simulink library "medusa5h1_stereo"  (R2022b)
settings: Solver=VariableStepAuto  StartTime=0.0  StopTime=10.0  RelTol=1e-3
values from neighbouring files (symbols this model uses):
  MedusaConfig = struct('BandSplitConfig', BandSplitConfig,                            'DRFDPConfig', DRFDPConfig,                            'FRFDPConfig', FRFDPConfig,                            'SurroundConfig', SurroundConfig,                            'MSConfig', MSConfig,                            'PremixConfig', PremixConfig.Stereo,                            'PremixTune', PremixTune.Stereo,               ...(+1303 chars)    [medusa5h1_init.m]
undefined symbols (not defined in the file or in its folder): Config, MedusaBTC, Row, VLSConfig
libraries: TuneVar x25, MedusaDelays x19, FeaturePath x15, RTC x6, MedusaCaeEnable x4, MedusaDrHoligramEq x4, TOP x4, BassManager x2, StateVar x2, TrebleBoost x2, dspstat3 x2, MedusaBandSplit x2
(part 2 of 2)

== system medusa5h1_stereo/Medusa + Holigram/Medusa5H1 Part 5/Triggered Subsystem ==
  Trigger : TriggerPort  TriggerType=function-call  VariantControl=(inherit)
  Constant : Constant  Value=0
  Data Store Write : DataStoreWrite  DataStoreName=MedusaOverheadHoligramEnable  IndexOptions=Index vector (dialog)  Indices=1  OutputSizes=1
  wires:
  Constant/1 -> Data Store Write/1

== system medusa5h1_stereo/Medusa + Holigram/Medusa5H1 Part 6/Speaker Delay Tune ==
  Output Delay Translation with Headrest : MedusaDelays/HeadrestOutputDelayTranslation  Config=ConfigBTC.HeadrestOutputDelayTranslation
  TOP3 : TOP/TOP  TriggerInit=[645 305 895 365]  TopName=FRSpeakerDelay  DataTypeOut=int32  BankNumber=0  PreOverlay=false  PostOverlay=false  Role=Automatic
      settings: SourceProductName=Bose Talaria
  TOP5 : TOP/TOP  TriggerInit=[645 155 895 215]  TopName=DRSpeakerDelay  DataTypeOut=int32  BankNumber=0  PreOverlay=false  PostOverlay=false  Role=Automatic
      settings: SourceProductName=Bose Talaria
  Tune Variable : TuneVar/TuneVar  TuneName=HeadrestDrvSpeakerDelaySamples  SpecifyMaxSize=off  VariableDim=1 (Row)  MaxSize=[1 1]  TunabilityNumber=1  MinValue=[]  MaxValue=[]  TriggerInit=[20 195 245 245]  MaskValue=[0]
      settings: SourceProductName=Bose Talaria
  Tune Variable1 : TuneVar/TuneVar  TuneName=NonHeadrestSpeakerDelaySamples  SpecifyMaxSize=off  VariableDim=1 (Row)  MaxSize=[]  TunabilityNumber=1  MinValue=[]  MaxValue=[]  TriggerInit=[20 120 245 170]  MaskValue=HRDelayConfig.DRNonHRDelay
      settings: SourceProductName=Bose Talaria
  Tune Variable4 : TuneVar/TuneVar  TuneName=HeadrestPaxSpeakerDelaySamples  SpecifyMaxSize=off  VariableDim=1 (Row)  MaxSize=[1 1]  TunabilityNumber=1  MinValue=[]  MaxValue=[]  TriggerInit=[20 270 245 320]  MaskValue=[0]
      settings: SourceProductName=Bose Talaria
  Tune Variable5 : TuneVar/TuneVar  TuneName=FRHoligramDelaySamples  SpecifyMaxSize=off  VariableDim=1 (Row)  MaxSize=[]  TunabilityNumber=1  MinValue=[]  MaxValue=[]  TriggerInit=[20 345 245 395]  MaskValue=HRDelayConfig.FRSpkrDelay
      settings: SourceProductName=Bose Talaria
  DRSpeakerDelay : Outport
  FRSpeakerDelay : Outport  Port=2
  wires:
  TOP5/1 -> DRSpeakerDelay/1  "DRSpeakerDelay"
  TOP3/1 -> FRSpeakerDelay/1  "FRSpeakerDelay"
  Tune Variable1/1 -> Output Delay Translation with Headrest/1  "NonHeadrestSpeakerDelaySamples"
  Tune Variable/1 -> Output Delay Translation with Headrest/2  "HeadrestDrvSpeakerDelaySamples"
  Tune Variable4/1 -> Output Delay Translation with Headrest/3  "HeadrestPaxSpeakerDelaySamples"
  Tune Variable5/1 -> Output Delay Translation with Headrest/4  "FRHoligramDelaySamples"
  Output Delay Translation with Headrest/1 -> TOP5/1
  Output Delay Translation with Headrest/2 -> TOP3/1

== system medusa5h1_stereo/Medusa5H1 Stereo/Medusa5H1 Part 1/CAE Treble Boost ==
  note: 1) Add Subsystem or Model blocks as valid variant choices.
      | 2) You cannot connect blocks at this level. At simulation, connectivity is automatically
      | determined, based on the active variant and port name matching.
  AudioIn : Inport
  Audio Passthrough : Subsystem  VariantControl=include_CAE == 0
  CAE Treble Boost : Subsystem  VariantControl=include_CAE == 1
  Out : Outport
  CAEEnable : Outport  Port=2

== system medusa5h1_stereo/Medusa5H1 Stereo/Medusa5H1 Part 2/Alignment Delay ==
  LRhp : Inport
  Full-rate Alignment Delay Translation : MedusaDelays/MedusaFullRateAlignmentDelayTranslation  Config=Config.TrebleDelayTranslation
  Treble Delay : MedusaDelays/MedusaAlignmentDelay  Config=Config.TrebleDelay
  Tune Variable1 : TuneVar/TuneVar  TuneName=DeciRateNearWiggleFilterDelaySamples  SpecifyMaxSize=off  VariableDim=1 (Row)  MaxSize=[1 1]  TunabilityNumber=1  MinValue=[]  MaxValue=[]  TriggerInit=[-55 450 110 500]  MaskValue=Config.TrebleDelayTranslation.DefaultTuning.DeciRateNearWiggleDelay
      settings: SourceProductName=Bose Talaria
  Tune Variable4 : TuneVar/TuneVar  TuneName=DeciRateWiggleFilterDelaySamples  SpecifyMaxSize=off  VariableDim=1 (Row)  MaxSize=[1 1]  TunabilityNumber=1  MinValue=[]  MaxValue=[]  TriggerInit=[-55 385 110 435]  MaskValue=Config.TrebleDelayTranslation.DefaultTuning.DeciRateWiggleDelay
      settings: SourceProductName=Bose Talaria
  Tune Variable5 : TuneVar/TuneVar  TuneName=HoligramFilterAlignmentDelaySamples  SpecifyMaxSize=off  VariableDim=1 (Row)  MaxSize=[1 1]  TunabilityNumber=1  MinValue=[]  MaxValue=[]  TriggerInit=[-55 515 110 565]  MaskValue=Config.TrebleDelayTranslation.DefaultTuning.HoligramDelay
      settings: SourceProductName=Bose Talaria
  LRtreble : Outport
  wires:
  [TrebleDelay] -> Treble Delay/2
  Tune Variable4/1 -> Full-rate Alignment Delay Translation/1  "DeciRateWiggleFilterDelaySamples"
  Full-rate Alignment Delay Translation/1 -> [TrebleDelay]
  Treble Delay/1 -> LRtreble/1  "LRtreble"
  LRhp/1 -> Treble Delay/1
  Tune Variable5/1 -> Full-rate Alignment Delay Translation/3  "HoligramFilterAlignmentDelaySamples"
  Tune Variable1/1 -> Full-rate Alignment Delay Translation/2  "DeciRateNearWiggleFilterDelaySamples"

== system medusa5h1_stereo/Medusa5H1 Stereo/Medusa5H1 Part 3/Bypass ==
  Action Port : ActionPort
  Constant : Constant  Value=zeros(config.PremixConfig.frame_size, config.PremixConfig.NumPremixOut)  OutDataTypeStr=single
  Constant1 : Constant  Value=Config.DefaultFullRateMixerOutput  OutDataTypeStr=single
  PremixOut : Outport  VectorParamsAs1DForOutWhenUnconnected=off
  FRMixerOut : Outport  Port=2  VectorParamsAs1DForOutWhenUnconnected=off
  wires:
  Constant/1 -> PremixOut/1
  Constant1/1 -> FRMixerOut/1

== system medusa5h1_stereo/Medusa5H1 Stereo/Medusa5H1 Part 3/Enable State Write ==
  Trigger : TriggerPort  TriggerType=function-call  VariantControl=Variant  PortDimensions=1
  Constant : Constant  Value=0  OutDataTypeStr=uint32
  Data Store Write : DataStoreWrite  DataStoreName=MedusaPostUpmixEnable  IndexOptions=Index vector (dialog)  Indices=1  OutputSizes=1
  wires:
  Constant/1 -> Data Store Write/1

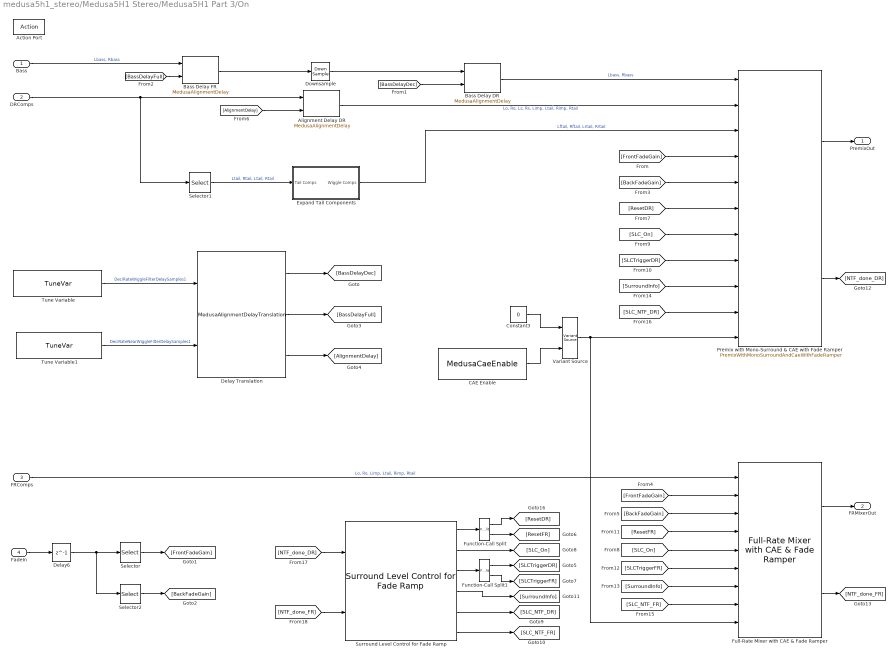
== system medusa5h1_stereo/Medusa5H1 Stereo/Medusa5H1 Part 3/On ==
  Bass : Inport  OutDataTypeStr=single
  DRComps : Inport  Port=2  OutDataTypeStr=single
  FRComps : Inport  Port=3  OutDataTypeStr=single
  FadeIn : Inport  Port=4  OutDataTypeStr=single
  Action Port : ActionPort
  Alignment Delay DR : MedusaDelays/MedusaAlignmentDelay  Config=Config.MidrangeDelay
  Bass Delay DR : MedusaDelays/MedusaAlignmentDelay  Config=Config.DeciRateBassDelay
  Bass Delay FR : MedusaDelays/MedusaAlignmentDelay  Config=Config.FullRateBassDelay
  CAE Enable : MedusaCaeEnable/MedusaCaeEnable  Config=Config.PremixCaeEnable  MaskMessageName=PremixCAEEnable
  Constant3 : Constant  Value=0  OutDataTypeStr=int32  SampleTime=-1
  Delay Translation : MedusaDelays/MedusaAlignmentDelayTranslation  Config=Config.AlignmentDelayTranslation
  Delay6 : Delay  DelayLength=1
  Downsample : DownSample  N=4
  Expand Tail Components : Subsystem  TreatAsAtomicUnit=on  RTWFileName=MedusaExpandTailComps
      settings: RTWSystemCode=Nonreusable function  RTWFileNameOpts=User specified  FunctionWithSeparateData=on
  Full-Rate Mixer with CAE & Fade Ramper : MedusaFullRateMixer/Full-Rate Mixer with CAE & Fade Ramper  MedusaFRMConfig=config.FRMConfig  MedusaFRMTune=config.FRMTune
  Function-Call Split : FunctionCallSplit  IconShape=distinctive  NumOutputPorts=2  OutputPortLayout=default
  Function-Call Split1 : FunctionCallSplit  IconShape=distinctive  NumOutputPorts=2  OutputPortLayout=default
  Premix with Mono-Surround & CAE with Fade Ramper : MedusaPremix/PremixWithMonoSurroundAndCaeWithFadeRamper  MedusaPremixConfig=config.PremixConfig  MedusaPremixTune=config.PremixTune  MSConfig=config.MSConfig
  Selector : Selector  NumberOfDimensions=2  InputPortWidth=2  IndexOptions=Index vector (dialog),Index vector (dialog)  Indices=1,1  OutputSizes=1,1
  Selector1 : Selector  NumberOfDimensions=2  InputPortWidth=3  IndexOptions=Select all,Index vector (dialog)  Indices=[1 3],[6 8 6 8]  OutputSizes=1,1
  Selector2 : Selector  NumberOfDimensions=2  InputPortWidth=2  IndexOptions=Index vector (dialog),Index vector (dialog)  Indices=1,2  OutputSizes=1,1
  Surround Level Control for Fade Ramp : MedusaSurroundLevelControl/Surround Level Control for Fade Ramp  SurroundConfig=config.SurroundConfig
  Tune Variable : TuneVar/TuneVar  TuneName=DeciRateWiggleFilterDelaySamples1  SpecifyMaxSize=off  VariableDim=1 (Row)  MaxSize=[1 1]  TunabilityNumber=1  MinValue=[]  MaxValue=[]  TriggerInit=[-70 585 100 635]  MaskValue=Config.AlignmentDelayTranslation.DefaultTuning.DeciRateWiggleDelay
      settings: SourceProductName=Bose Talaria
  Tune Variable1 : TuneVar/TuneVar  TuneName=DeciRateNearWiggleFilterDelaySamples1  SpecifyMaxSize=off  VariableDim=1 (Row)  MaxSize=[1 1]  TunabilityNumber=1  MinValue=[]  MaxValue=[]  TriggerInit=[-65 705 100 755]  MaskValue=Config.AlignmentDelayTranslation.DefaultTuning.DeciRateNearWiggleDelay
      settings: SourceProductName=Bose Talaria
  Variant Source : VariantSource
  PremixOut : Outport  VectorParamsAs1DForOutWhenUnconnected=off
  FRMixerOut : Outport  Port=2  VectorParamsAs1DForOutWhenUnconnected=off
  wires:
  Selector/1 -> [FrontFadeGain]
  Delay6/1 -> Selector/1, Selector2/1
  Selector2/1 -> [BackFadeGain]
  FadeIn/1 -> Delay6/1
  Bass Delay FR/1 -> Downsample/1
  Alignment Delay DR/1 -> Premix with Mono-Surround & CAE with Fade Ramper/2  "Lo, Ro, Ls, Rs, Limp, Ltail, Rimp, Rtail"
  DRComps/1 -> Selector1/1, Alignment Delay DR/1
  Selector1/1 -> Expand Tail Components/1(Tail Comps)  "Ltail, Rtail, Ltail, Rtail"
  Bass/1 -> Bass Delay FR/1  "Lbass, Rbass"
  Expand Tail Components/1(Wiggle Comps) -> Premix with Mono-Surround & CAE with Fade Ramper/3  "Lftail, Rftail, Lrtail, Rrtail"
  [BackFadeGain] -> Premix with Mono-Surround & CAE with Fade Ramper/5
  [FrontFadeGain] -> Full-Rate Mixer with CAE & Fade Ramper/2
  Premix with Mono-Surround & CAE with Fade Ramper/1 -> PremixOut/1
  [BackFadeGain] -> Full-Rate Mixer with CAE & Fade Ramper/3
  Full-Rate Mixer with CAE & Fade Ramper/1 -> FRMixerOut/1
  [FrontFadeGain] -> Premix with Mono-Surround & CAE with Fade Ramper/4
  Delay Translation/3 -> [AlignmentDelay]
  Delay Translation/2 -> [BassDelayFull]
  Delay Translation/1 -> [BassDelayDec]
  Tune Variable/1 -> Delay Translation/1  "DeciRateWiggleFilterDelaySamples1"
  [BassDelayFull] -> Bass Delay FR/2
  [AlignmentDelay] -> Alignment Delay DR/2
  Bass Delay DR/1 -> Premix with Mono-Surround & CAE with Fade Ramper/1  "Lbass, Rbass"
  [BassDelayDec] -> Bass Delay DR/2
  Downsample/1 -> Bass Delay DR/1
  FRComps/1 -> Full-Rate Mixer with CAE & Fade Ramper/1  "Lo, Ro, Limp, Ltail, Rimp, Rtail"
  Surround Level Control for Fade Ramp/1 -> Function-Call Split/1
  Surround Level Control for Fade Ramp/3 -> Function-Call Split1/1
  Function-Call Split/1 -> [ResetDR]
  Function-Call Split/2 -> [ResetFR]
  Function-Call Split1/1 -> [SLCTriggerDR]
  Function-Call Split1/2 -> [SLCTriggerFR]
  Surround Level Control for Fade Ramp/2 -> [SLC_On]
  Surround Level Control for Fade Ramp/4 -> [SurroundInfo]
  Surround Level Control for Fade Ramp/5 -> [SLC_NTF_DR]
  Surround Level Control for Fade Ramp/6 -> [SLC_NTF_FR]
  [ResetFR] -> Full-Rate Mixer with CAE & Fade Ramper/4
  Premix with Mono-Surround & CAE with Fade Ramper/2 -> [NTF_done_DR]
  [NTF_done_FR] -> Surround Level Control for Fade Ramp/2
  [NTF_done_DR] -> Surround Level Control for Fade Ramp/1
  [ResetDR] -> Premix with Mono-Surround & CAE with Fade Ramper/6
  [SLC_NTF_DR] -> Premix with Mono-Surround & CAE with Fade Ramper/10
  [SurroundInfo] -> Premix with Mono-Surround & CAE with Fade Ramper/9
  [SLCTriggerDR] -> Premix with Mono-Surround & CAE with Fade Ramper/8
  [SLC_On] -> Premix with Mono-Surround & CAE with Fade Ramper/7
  Constant3/1 -> Variant Source/1
  CAE Enable/1 -> Variant Source/2
  Variant Source/1 -> Premix with Mono-Surround & CAE with Fade Ramper/11, Full-Rate Mixer with CAE & Fade Ramper/9
  [SLC_NTF_FR] -> Full-Rate Mixer with CAE & Fade Ramper/8
  [SurroundInfo] -> Full-Rate Mixer with CAE & Fade Ramper/7
  [SLCTriggerFR] -> Full-Rate Mixer with CAE & Fade Ramper/6
  [SLC_On] -> Full-Rate Mixer with CAE & Fade Ramper/5
  Full-Rate Mixer with CAE & Fade Ramper/2 -> [NTF_done_FR]
  Tune Variable1/1 -> Delay Translation/2  "DeciRateNearWiggleFilterDelaySamples1"

== system medusa5h1_stereo/Medusa5H1 Stereo/Medusa5H1 Part 4/Bypass ==
  Action Port : ActionPort
  Constant : Constant  Value=MedusaConfig.outputDefault  OutDataTypeStr=single
  IsStereo : Outport  VectorParamsAs1DForOutWhenUnconnected=off
  wires:
  Constant/1 -> IsStereo/1

== system medusa5h1_stereo/Medusa5H1 Stereo/Medusa5H1 Part 4/Enable State Write ==
  Trigger : TriggerPort  TriggerType=function-call  VariantControl=Variant  PortDimensions=1
  Constant : Constant  Value=0  OutDataTypeStr=uint32
  Data Store Write : DataStoreWrite  DataStoreName=MedusaHoligramEnable  IndexOptions=Index vector (dialog)  Indices=1  OutputSizes=1
  wires:
  Constant/1 -> Data Store Write/1

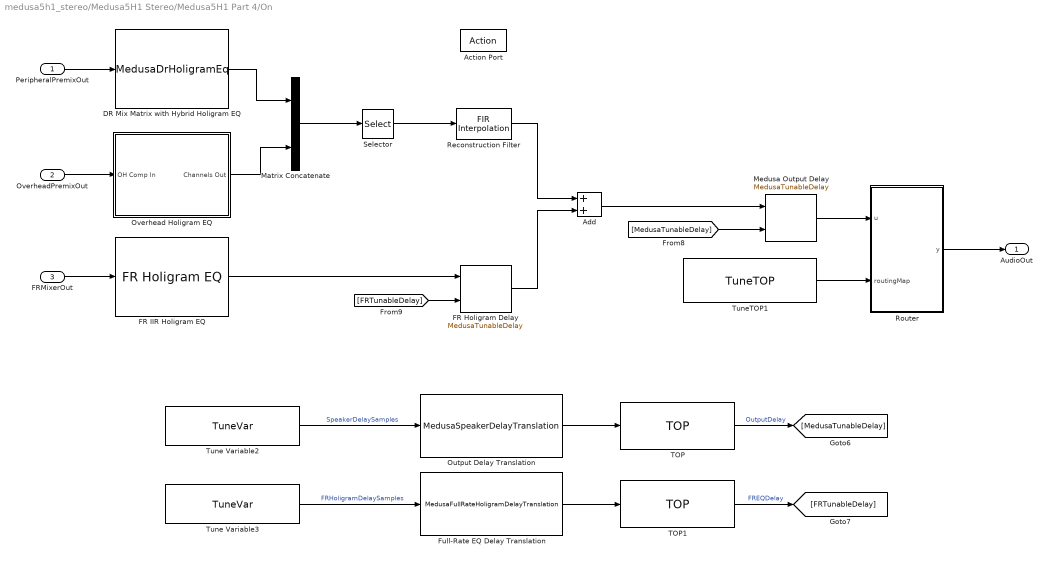
== system medusa5h1_stereo/Medusa5H1 Stereo/Medusa5H1 Part 4/On ==
  PeripheralPremixOut : Inport  OutDataTypeStr=single
  OverheadPremixOut : Inport  Port=2  OutDataTypeStr=single
  FRMixerOut : Inport  Port=3  OutDataTypeStr=single
  Action Port : ActionPort
  Add : Sum
  DR Mix Matrix with Hybrid Holigram EQ : MedusaDrHoligramEq/MedusaDrHoligramEq  Config=Config.PeripheralHoligramEq.HoligramEq
  FR Holigram Delay : MedusaDelays/MedusaTunableDelay  Config=Config.FullRateHoligramDelay
  FR IIR Holigram EQ : MedusaFRHoligramEQ/FR Holigram EQ  configStruct=config.HoligramEQConfig
  Full-Rate EQ Delay Translation : MedusaDelays/MedusaFullRateHoligramDelayTranslation  Config=Config.FullRateHoligramDelayTranslation
  Matrix Concatenate : Concatenate  Mode=Multidimensional array  ConcatenateDimension=2
  Medusa Output Delay : MedusaDelays/MedusaTunableDelay  Config=Config.SpeakerDelay
  Output Delay Translation : MedusaDelays/MedusaSpeakerDelayTranslation  Config=Config.SpeakerDelayTranslation
  Overhead Holigram EQ : Subsystem  Variant=on
  Reconstruction Filter : dspmlti4/FIR Interpolation  FilterSource=Dialog parameters  PrivateCoeffs=0  h=config.BandSplitConfig.upfir  L=config.BandSplitConfig.D  FilterObject=FINTERP  InputProcessing=Columns as channels (frame based)  framing=Enforce single-rate processing  outputBufInitCond=0  roundingMode=Floor  overflowMode=off  firstCoeffDataTypeStr=Inherit: Same word length as input  firstCoeffMin=[]  firstCoeffMax=[]  firstCoeffLastDataTypeStr=Inherit: Same word length as input  outputDataTypeStr=Inherit: Same as accumulator  outputMin=[]  outputMax=[]  outputLastDataTypeStr=Inherit: Same as accumulator
  Router : MATLAB Function  TreatAsAtomicUnit=on
  Selector : Selector  NumberOfDimensions=2  InputPortWidth=3  IndexOptions=Select all,Index vector (dialog)  Indices=[1 3],1:config.numMedusaOut  OutputSizes=1,1
  TOP : TOP/TOP  TriggerInit=[2225 900 2370 960]  TopName=OutputDelay  DataTypeOut=int32  BankNumber=0  PreOverlay=false  PostOverlay=false  Role=Automatic
      settings: SourceProductName=Bose Talaria
  TOP1 : TOP/TOP  TriggerInit=[2225 1000 2370 1060]  TopName=FREQDelay  DataTypeOut=int32  BankNumber=0  PreOverlay=false  PostOverlay=false  Role=Automatic
      settings: SourceProductName=Bose Talaria
  Tune Variable2 : TuneVar/TuneVar  TuneName=SpeakerDelaySamples  SpecifyMaxSize=off  VariableDim=1 (Row)  MaxSize=[]  TunabilityNumber=1  MinValue=[]  MaxValue=[]  TriggerInit=[1645 905 1815 955]  MaskValue=Config.Get(@Config.SpeakerDelayTranslation.DefaultTuning.SpeakerDelay)
      settings: SourceProductName=Bose Talaria
  Tune Variable3 : TuneVar/TuneVar  TuneName=FRHoligramDelaySamples  SpecifyMaxSize=off  VariableDim=1 (Row)  MaxSize=[]  TunabilityNumber=1  MinValue=[]  MaxValue=[]  TriggerInit=[1645 1005 1815 1055]  MaskValue=Config.Get(@Config.FullRateHoligramDelayTranslation.DefaultTuning.FullRateHoligramDelay)
      settings: SourceProductName=Bose Talaria
  TuneTOP1 : TuneVar/TuneTOP  TriggerInit=[2305 717 2475 773]  TopName=RoutingMap  TuneName=RoutingMap  DataTypeOut=single  TunabilityNumber=1  MinValue=[]  MaxValue=[]  BankNumber=0  PreOverlay=false  PostOverlay=false  UseSameName=on  MaskValue=config.routingMapDefault
      settings: SourceProductName=Bose Talaria
  AudioOut : Outport  VectorParamsAs1DForOutWhenUnconnected=off
  wires:
  FR IIR Holigram EQ/1 -> FR Holigram Delay/1
  Medusa Output Delay/1 -> Router/1(u)
  FR Holigram Delay/1 -> Add/2
  Add/1 -> Medusa Output Delay/1
  TuneTOP1/1 -> Router/2(routingMap)
  Reconstruction Filter/1 -> Add/1
  Router/1(y) -> AudioOut/1
  Tune Variable2/1 -> Output Delay Translation/1  "SpeakerDelaySamples"
  TOP/1 -> [MedusaTunableDelay]  "OutputDelay"
  Tune Variable3/1 -> Full-Rate EQ Delay Translation/1  "FRHoligramDelaySamples"
  [MedusaTunableDelay] -> Medusa Output Delay/2
  [FRTunableDelay] -> FR Holigram Delay/2
  Output Delay Translation/1 -> TOP/1
  Full-Rate EQ Delay Translation/1 -> TOP1/1
  TOP1/1 -> [FRTunableDelay]  "FREQDelay"
  PeripheralPremixOut/1 -> DR Mix Matrix with Hybrid Holigram EQ/1
  FRMixerOut/1 -> FR IIR Holigram EQ/1
  OverheadPremixOut/1 -> Overhead Holigram EQ/1(OH Comp In)
  Overhead Holigram EQ/1(Channels Out) -> Matrix Concatenate/2
  Matrix Concatenate/1 -> Selector/1
  DR Mix Matrix with Hybrid Holigram EQ/1 -> Matrix Concatenate/1
  Selector/1 -> Reconstruction Filter/1

== system medusa5h1_stereo/Medusa + Holigram/Medusa5H1 Part 1/CAE Treble Boost/Audio Passthrough ==
  AudioIn : Inport
  Constant : Constant  Value=0  OutDataTypeStr=int32  SampleTime=-1
  Constant3 : Constant  Value=0  OutDataTypeStr=int32  SampleTime=-1
  Target StateVar : StateVar/TargetStateVar  TriggerInit=[235 166 375 234]  TspName=DummyState  StateName=DummyState  UseSameName=on  IfdefMacro=[]
      settings: SourceProductName=Bose Talaria
  Terminator : Terminator
  TuneTOP : TuneVar/TuneTOP  TriggerInit=[50 262 220 318]  TopName=DummyTune  TuneName=DummyTune  DataTypeOut=single  TunabilityNumber=1  MinValue=[]  MaxValue=[]  BankNumber=0  PreOverlay=false  PostOverlay=false  UseSameName=on  MaskValue=[1]
      settings: SourceProductName=Bose Talaria
  Out : Outport
  CAEEnable : Outport  Port=2
  wires:
  AudioIn/1 -> Out/1
  TuneTOP/1 -> Terminator/1
  Constant/1 -> Target StateVar/1
  Constant3/1 -> CAEEnable/1

== system medusa5h1_stereo/Medusa + Holigram/Medusa5H1 Part 1/CAE Treble Boost/CAE Treble Boost ==
  AudioIn : Inport
  CAE Enable : MedusaCaeEnable/MedusaCaeEnable  Config=Config.CaeEnable  MaskMessageName=CAEEnable
  Treble Boost : TrebleBoost/TrebleBoostStereo  Config=Config.TrebleBoost
  Tune Variable4 : TuneVar/TuneVar  Description=|  TuneName=SurroundOn  SpecifyMaxSize=off  VariableDim=1 (Row)  MaxSize=[1 1]  TunabilityNumber=1  MinValue=[]  MaxValue=[]  TriggerInit=[-50 35 120 85]  MaskValue=2
      | General surround control parameter
      | STEREO_MODE = 0
      | SURROUND_PASSTHRU_MODE = 1
      | MEDUSA_2_CHANNEL_MODE = 2
      | MEDUSA_5_1_MODE = 3
      settings: SourceProductName=Bose Talaria
  Out : Outport
  CAEEnable : Outport  Port=2
  wires:
  CAE Enable/1 -> Treble Boost/3, CAEEnable/1
  Tune Variable4/1 -> Treble Boost/2  "SurroundOn"
  AudioIn/1 -> Treble Boost/1
  Treble Boost/1 -> Out/1

== system medusa5h1_stereo/Medusa + Holigram/Medusa5H1 Part 3/On/Delay Tuning ==
  Delay Translation : MedusaDelays/MedusaAlignmentDelayTranslation  Config=ConfigBTC.AlignmentDelayTranslation
  Tune Variable : TuneVar/TuneVar  TuneName=DeciRateWiggleFilterDelaySamples1  SpecifyMaxSize=off  VariableDim=1 (Row)  MaxSize=[1 1]  TunabilityNumber=1  MinValue=[]  MaxValue=[]  TriggerInit=[-115 25 55 75]  MaskValue=ConfigBTC.AlignmentDelayTranslation.DefaultTuning.DeciRateWiggleDelay
      settings: SourceProductName=Bose Talaria
  Tune Variable1 : TuneVar/TuneVar  TuneName=DeciRateNearWiggleFilterDelaySamples1  SpecifyMaxSize=off  VariableDim=1 (Row)  MaxSize=[1 1]  TunabilityNumber=1  MinValue=[]  MaxValue=[]  TriggerInit=[-115 87 55 133]  MaskValue=ConfigBTC.AlignmentDelayTranslation.DefaultTuning.DeciRateNearWiggleDelay
      settings: SourceProductName=Bose Talaria
  Out1 : Outport
  Out2 : Outport  Port=2
  Out3 : Outport  Port=3
  wires:
  Tune Variable/1 -> Delay Translation/1  "DeciRateWiggleFilterDelaySamples1"
  Delay Translation/2 -> Out2/1
  Delay Translation/1 -> Out1/1
  Delay Translation/3 -> Out3/1
  Tune Variable1/1 -> Delay Translation/2  "DeciRateNearWiggleFilterDelaySamples1"

== system medusa5h1_stereo/Medusa + Holigram/Medusa5H1 Part 3/On/Expand Tail Components ==
  Tail Comps : Inport
  Constant : Constant  Value=[0 1 2 3]  OutDataTypeStr=single  SampleTime=-1
  Tail Component EQ : PooliirLib/PooliirwithNonTrivialTranslations  maxNumStages=config.tailCompEQ.maxNumStages  numStages=config.tailCompEQ.numStages  sosCoefficients=config.tailCompEQ.coeffs  alias='Default'  variantType='Hexagon'  FeatureName=tailCompEQ
  TuneTOP : TuneVar/TuneTOP  TriggerInit=[265 167 435 223]  TopName=WiggleFilter  TuneName=WiggleFilter  DataTypeOut=single  TunabilityNumber=1  MinValue=[]  MaxValue=[]  BankNumber=0  PreOverlay=false  PostOverlay=false  UseSameName=on  MaskValue=config.wiggleFilterDefault
      settings: SourceProductName=Bose Talaria
  Wiggle Filters : FirEven/FirEven  Config=config.TailCompFirEvenSettings
      settings: SourceProductName=Bose Blocklib
  Wiggle Comps : Outport  VectorParamsAs1DForOutWhenUnconnected=off
  wires:
  [wiggleFilter] -> Wiggle Filters/2
  Wiggle Filters/1 -> Tail Component EQ/1  "Lftail, Rftail, Lrtail, Rrtail"
  TuneTOP/1 -> [wiggleFilter]
  Constant/1 -> Wiggle Filters/3
  Tail Component EQ/1 -> Wiggle Comps/1
  Tail Comps/1 -> Wiggle Filters/1  "Ltail, Rtail, Ltail, Rtail"

== system medusa5h1_stereo/Medusa + Holigram/Medusa5H1 Part 3/On/Full-rate Mixer ==
  Upmix In : Inport
  CAE Control : Inport  Port=2
  Full-Rate Mixer with CAE & Fade Ramper : MedusaFullRateMixer/Full-Rate Mixer with CAE & Fade Ramper  MedusaFRMConfig=config.FRMConfig  MedusaFRMTune=config.FRMTune
  Out1 : Outport
  tag scope: NTFDone2=global
  wires:
  Upmix In/1 -> Full-Rate Mixer with CAE & Fade Ramper/1
  Full-Rate Mixer with CAE & Fade Ramper/1 -> Out1/1
  [FrontFadeGain] -> Full-Rate Mixer with CAE & Fade Ramper/2
  [SLCReset2] -> Full-Rate Mixer with CAE & Fade Ramper/4
  Full-Rate Mixer with CAE & Fade Ramper/2 -> [NTFDone2]
  [SLCTrigger2] -> Full-Rate Mixer with CAE & Fade Ramper/6
  [SurroundInfo] -> Full-Rate Mixer with CAE & Fade Ramper/7
  [BackFadeGain] -> Full-Rate Mixer with CAE & Fade Ramper/3
  [NTFCheck2] -> Full-Rate Mixer with CAE & Fade Ramper/8
  [SLC_On] -> Full-Rate Mixer with CAE & Fade Ramper/5
  CAE Control/1 -> Full-Rate Mixer with CAE & Fade Ramper/9

== system medusa5h1_stereo/Medusa + Holigram/Medusa5H1 Part 3/On/Premix ==
  Bass In : Inport
  Upmix In : Inport  Port=2
  Wiggle In : Inport  Port=3
  CAE Control : Inport  Port=4
  Premix with Mono-Surround & CAE with Fade Ramper : MedusaPremix/PremixWithMonoSurroundAndCaeWithFadeRamper  MedusaPremixConfig=config.PremixConfig  MedusaPremixTune=config.PremixTune  MSConfig=config.MSConfig
      settings: LibrarySourceBlock=MedusaPremix/Premix with Mono-Surround & CAE with Fade Ramper
  Out1 : Outport
  tag scope: NTFDone1=global
  wires:
  Bass In/1 -> Premix with Mono-Surround & CAE with Fade Ramper/1
  [SurroundInfo] -> Premix with Mono-Surround & CAE with Fade Ramper/9
  [FrontFadeGain] -> Premix with Mono-Surround & CAE with Fade Ramper/4
  [SLCTrigger1] -> Premix with Mono-Surround & CAE with Fade Ramper/8
  [SLCReset1] -> Premix with Mono-Surround & CAE with Fade Ramper/6
  [NTFCheck1] -> Premix with Mono-Surround & CAE with Fade Ramper/10
  [BackFadeGain] -> Premix with Mono-Surround & CAE with Fade Ramper/5
  Wiggle In/1 -> Premix with Mono-Surround & CAE with Fade Ramper/3
  Upmix In/1 -> Premix with Mono-Surround & CAE with Fade Ramper/2
  Premix with Mono-Surround & CAE with Fade Ramper/2 -> [NTFDone1]
  Premix with Mono-Surround & CAE with Fade Ramper/1 -> Out1/1
  CAE Control/1 -> Premix with Mono-Surround & CAE with Fade Ramper/11
  [SLC_On] -> Premix with Mono-Surround & CAE with Fade Ramper/7

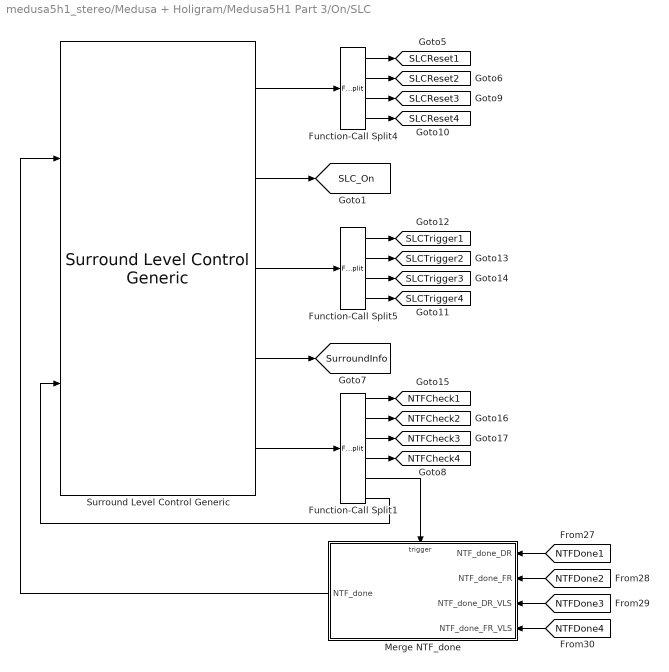
== system medusa5h1_stereo/Medusa + Holigram/Medusa5H1 Part 3/On/SLC ==
  Function-Call Split1 : FunctionCallSplit  IconShape=distinctive  NumOutputPorts=6  OutputPortLayout=default
  Function-Call Split4 : FunctionCallSplit  IconShape=distinctive  NumOutputPorts=4  OutputPortLayout=default
  Function-Call Split5 : FunctionCallSplit  IconShape=distinctive  NumOutputPorts=4  OutputPortLayout=default
  Merge NTF_done : Subsystem
  Surround Level Control Generic : MedusaSurroundLevelControl/Surround Level Control Generic  SurroundConfig=config.SurroundConfig
  tag scope: NTFCheck1=global, NTFCheck2=global, NTFCheck3=global, NTFCheck4=global, SLCReset1=global, SLCReset2=global, SLCReset3=global, SLCReset4=global, SLCTrigger1=global, SLCTrigger2=global, SLCTrigger3=global, SLCTrigger4=global, SLC_On=global, SurroundInfo=global
  wires:
  Function-Call Split1/3 -> [NTFCheck3]
  Surround Level Control Generic/1 -> Function-Call Split4/1
  [NTFDone1] -> Merge NTF_done/1(NTF_done_DR)
  Function-Call Split1/1 -> [NTFCheck1]
  Function-Call Split1/2 -> [NTFCheck2]
  Function-Call Split5/2 -> [SLCTrigger2]
  Function-Call Split1/4 -> [NTFCheck4]
  [NTFDone2] -> Merge NTF_done/2(NTF_done_FR)
  Function-Call Split4/2 -> [SLCReset2]
  Function-Call Split1/5 -> Merge NTF_done/Trigger
  [NTFDone4] -> Merge NTF_done/4(NTF_done_FR_VLS)
  Function-Call Split4/3 -> [SLCReset3]
  Function-Call Split5/4 -> [SLCTrigger4]
  Function-Call Split4/1 -> [SLCReset1]
  Surround Level Control Generic/4 -> [SurroundInfo]
  Surround Level Control Generic/3 -> Function-Call Split5/1
  Function-Call Split5/1 -> [SLCTrigger1]
  Function-Call Split5/3 -> [SLCTrigger3]
  Function-Call Split4/4 -> [SLCReset4]
  [NTFDone3] -> Merge NTF_done/3(NTF_done_DR_VLS)
  Merge NTF_done/1(NTF_done) -> Surround Level Control Generic/1
  Surround Level Control Generic/5 -> Function-Call Split1/1
  Surround Level Control Generic/2 -> [SLC_On]
  Function-Call Split1/6 -> Surround Level Control Generic/2

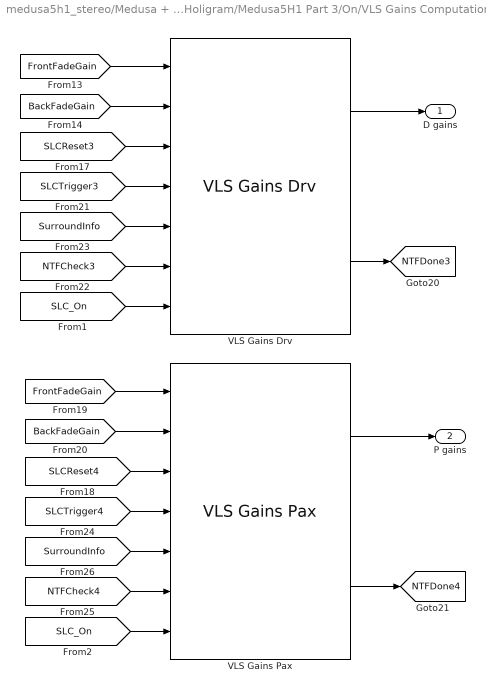
== system medusa5h1_stereo/Medusa + Holigram/Medusa5H1 Part 3/On/VLS Gains Computation ==
  VLS Gains Drv : VLSGains/VLS Gains Drv  configStruct=vlsConfigStruct.VLSGainsConfig  tuneStruct=vlsConfigStruct.VLSGainsTune  FeatureName=VLSDrvGains
  VLS Gains Pax : VLSGains/VLS Gains Pax  configStruct=vlsConfigStruct.VLSGainsConfig  tuneStruct=vlsConfigStruct.VLSGainsTune  FeatureName=VLSPaxGains
  D gains : Outport
  P gains : Outport  Port=2
  tag scope: NTFDone3=global, NTFDone4=global
  wires:
  [NTFCheck3] -> VLS Gains Drv/6
  [SLCReset3] -> VLS Gains Drv/3
  [BackFadeGain] -> VLS Gains Pax/2
  [SurroundInfo] -> VLS Gains Drv/5
  VLS Gains Pax/2 -> [NTFDone4]
  VLS Gains Drv/2 -> [NTFDone3]
  [SLCTrigger3] -> VLS Gains Drv/4
  [BackFadeGain] -> VLS Gains Drv/2
  [NTFCheck4] -> VLS Gains Pax/6
  [SurroundInfo] -> VLS Gains Pax/5
  [FrontFadeGain] -> VLS Gains Pax/1
  [SLCTrigger4] -> VLS Gains Pax/4
  [SLCReset4] -> VLS Gains Pax/3
  [FrontFadeGain] -> VLS Gains Drv/1
  VLS Gains Drv/1 -> D gains/1
  VLS Gains Pax/1 -> P gains/1
  [SLC_On] -> VLS Gains Drv/7
  [SLC_On] -> VLS Gains Pax/7

== system medusa5h1_stereo/Medusa + Holigram/Medusa5H1 Part 5/On/Overhead Holigram EQ ==
  OH Comp In : Inport
  Disable Overhead EQ : Subsystem  VariantControl=sys_defs.number_of_overhead_speaker_pairs == 0
  Enable Overhead EQ : Subsystem  VariantControl=sys_defs.number_of_overhead_speaker_pairs ~= 0
  Channels Out : Outport

== system medusa5h1_stereo/Medusa5H1 Stereo/Medusa5H1 Part 1/CAE Treble Boost/Audio Passthrough ==
  AudioIn : Inport
  Constant : Constant  Value=0  OutDataTypeStr=int32  SampleTime=-1
  Constant1 : Constant  Value=0  OutDataTypeStr=int32  SampleTime=-1
  Target StateVar : StateVar/TargetStateVar  TriggerInit=[235 151 375 219]  TspName=DummyState  StateName=DummyState  UseSameName=on  IfdefMacro=[]
      settings: SourceProductName=Bose Talaria
  Terminator : Terminator
  TuneTOP : TuneVar/TuneTOP  TriggerInit=[50 242 220 298]  TopName=DummyTune  TuneName=DummyTune  DataType=single  TunabilityNumber=1  MinValue=[]  MaxValue=[]  BankNumber=0  PreOverlay=false  PostOverlay=false  UseSameName=on  MaskValue=0
      settings: SourceProductName=Bose Talaria
  Out : Outport
  CAEEnable : Outport  Port=2
  wires:
  AudioIn/1 -> Out/1
  Constant/1 -> CAEEnable/1
  Constant1/1 -> Target StateVar/1
  TuneTOP/1 -> Terminator/1

== system medusa5h1_stereo/Medusa5H1 Stereo/Medusa5H1 Part 1/CAE Treble Boost/CAE Treble Boost ==
  AudioIn : Inport
  CAE Enable : MedusaCaeEnable/MedusaCaeEnable  Config=Config.CaeEnable  MaskMessageName=CAEEnable
  Treble Boost : TrebleBoost/TrebleBoostStereo  Config=Config.TrebleBoost
  Tune Variable4 : TuneVar/TuneVar  Description=|  TuneName=SurroundOn  SpecifyMaxSize=off  VariableDim=1 (Row)  MaxSize=[1 1]  TunabilityNumber=1  MinValue=[]  MaxValue=[]  TriggerInit=[-55 35 115 85]  MaskValue=2
      | General surround control parameter
      | STEREO_MODE = 0
      | SURROUND_PASSTHRU_MODE = 1
      | MEDUSA_2_CHANNEL_MODE = 2
      | MEDUSA_5_1_MODE = 3
      settings: SourceProductName=Bose Talaria
  Out : Outport
  CAEEnable : Outport  Port=2
  wires:
  Tune Variable4/1 -> Treble Boost/2  "SurroundOn"
  AudioIn/1 -> Treble Boost/1
  CAE Enable/1 -> Treble Boost/3, CAEEnable/1
  Treble Boost/1 -> Out/1

== system medusa5h1_stereo/Medusa5H1 Stereo/Medusa5H1 Part 3/On/Expand Tail Components ==
  Tail Comps : Inport
  Constant : Constant  Value=[0 1 2 3]  OutDataTypeStr=single  SampleTime=-1
  Tail Component EQ : PooliirLib/PooliirwithNonTrivialTranslations  maxNumStages=tailCompEQ.maxNumStages  numStages=tailCompEQ.numStages  sosCoefficients=tailCompEQ.coeffs  FeatureName=tailCompEQ
  TuneTOP : TuneVar/TuneTOP  TriggerInit=[265 167 435 223]  TopName=WiggleFilter  TuneName=WiggleFilter  DataType=single  TunabilityNumber=1  MinValue=[]  MaxValue=[]  BankNumber=0  PreOverlay=false  PostOverlay=false  UseSameName=on  MaskValue=config.wiggleFilterDefault
      settings: SourceProductName=Bose Talaria
  Wiggle Filters : FirEven/FirEven  Config=config.TailCompFirEvenSettings
      settings: SourceProductName=Bose Blocklib
  Wiggle Comps : Outport  VectorParamsAs1DForOutWhenUnconnected=off
  wires:
  [wiggleFilter] -> Wiggle Filters/2
  Wiggle Filters/1 -> Tail Component EQ/1  "Lftail, Rftail, Lrtail, Rrtail"
  TuneTOP/1 -> [wiggleFilter]
  Constant/1 -> Wiggle Filters/3
  Tail Component EQ/1 -> Wiggle Comps/1
  Tail Comps/1 -> Wiggle Filters/1  "Ltail, Rtail, Ltail, Rtail"

== system medusa5h1_stereo/Medusa5H1 Stereo/Medusa5H1 Part 4/On/Overhead Holigram EQ ==
  OH Comp In : Inport
  Disable Overhead EQ : Subsystem  VariantControl=sys_defs.number_of_overhead_speaker_pairs == 0
  Enable Overhead EQ : Subsystem  VariantControl=sys_defs.number_of_overhead_speaker_pairs ~= 0
  Channels Out : Outport

== system medusa5h1_stereo/Medusa + Holigram/Medusa5H1 Part 3/On/SLC/Merge NTF_done ==
  NTF_done_DR : Inport
  NTF_done_FR : Inport  Port=2
  NTF_done_DR_VLS : Inport  Port=3
  NTF_done_FR_VLS : Inport  Port=4
  Trigger : TriggerPort  TriggerType=function-call  VariantControl=Variant  PortDimensions=1
  AND : Logic  Inputs=4  IconShape=distinctive  AllPortsSameDT=off  OutDataTypeStr=boolean
  NTF_done : Outport  VectorParamsAs1DForOutWhenUnconnected=off
  wires:
  AND/1 -> NTF_done/1
  NTF_done_FR/1 -> AND/2
  NTF_done_DR/1 -> AND/1
  NTF_done_DR_VLS/1 -> AND/3
  NTF_done_FR_VLS/1 -> AND/4

== system medusa5h1_stereo/Medusa + Holigram/Medusa5H1 Part 5/On/Overhead Holigram EQ/Disable Overhead EQ ==
  OH Comp In : Inport
  Constant : Constant  Value=zeros(ConfigBTC.DeciRateFrameSize, 1)  VectorParams1D=off  OutDataTypeStr=single  SampleTime=-1
  Terminator : Terminator
  Channels Out : Outport
  wires:
  Constant/1 -> Channels Out/1
  OH Comp In/1 -> Terminator/1

== system medusa5h1_stereo/Medusa + Holigram/Medusa5H1 Part 5/On/Overhead Holigram EQ/Enable Overhead EQ ==
  OH Comp In : Inport
  DR Mix Matrix with Hybrid Holigram EQ : MedusaDrHoligramEq/MedusaDrHoligramEq  Config=ConfigBTC.OverheadHoligramEq.HoligramEq
  FeaturePath : FeaturePath/FeaturePath  FeatureName=Overhead  IsGroup=off  GroupNumber=-1  IsModule=off  TriggerInit=[10 -136 125 -29]
      settings: SourceProductName=Bose Talaria
  Channels Out : Outport
  wires:
  OH Comp In/1 -> DR Mix Matrix with Hybrid Holigram EQ/1
  DR Mix Matrix with Hybrid Holigram EQ/1 -> Channels Out/1

== system medusa5h1_stereo/Medusa5H1 Stereo/Medusa5H1 Part 4/On/Overhead Holigram EQ/Disable Overhead EQ ==
  OH Comp In : Inport
  Constant : Constant  Value=Config.DefaultOverheadHoligramEqOutput  OutDataTypeStr=single
  Terminator : Terminator
  Channels Out : Outport
  wires:
  Constant/1 -> Channels Out/1
  OH Comp In/1 -> Terminator/1

== system medusa5h1_stereo/Medusa5H1 Stereo/Medusa5H1 Part 4/On/Overhead Holigram EQ/Enable Overhead EQ ==
  OH Comp In : Inport
  DR Mix Matrix with Hybrid Holigram EQ : MedusaDrHoligramEq/MedusaDrHoligramEq  Config=Config.OverheadHoligramEq.HoligramEq
  FeaturePath : FeaturePath/FeaturePath  FeatureName=Overhead  IsGroup=off  GroupNumber=-1  IsModule=off  TriggerInit=[10 -136 125 -29]
      settings: SourceProductName=Bose Talaria
  Channels Out : Outport
  wires:
  OH Comp In/1 -> DR Mix Matrix with Hybrid Holigram EQ/1
  DR Mix Matrix with Hybrid Holigram EQ/1 -> Channels Out/1

== matlab function medusa5h1_stereo/Medusa5H1 Stereo/Medusa5H1 Part 4/On/Router ==
  data: u input; y output; routingMap input
function y = fcn(u, routingMap)

[frameSize, numIn] = size(u);
numOut = numel(routingMap);
y = coder.nullcopy(single(zeros(frameSize, numOut)));

for i = 1:numOut
    index = routingMap(i);
    if (index < 0) || (index >= numIn)
        y(:,i) = zeros(frameSize,1);
    else
        y(:,i) = u(:, index + 1); % add 1 for Matlab indexing
    end
end

== matlab function medusa5h1_stereo/MedusaPostHoligram/On/Router ==
  data: u input; y output; routingMap input
function y = fcn(u, routingMap)

[frameSize, numIn] = size(u);
numOut = numel(routingMap);
y = coder.nullcopy(single(zeros(frameSize, numOut)));

for i = 1:numOut
    index = routingMap(i);
    if (index < 0) || (index >= numIn)
        y(:,i) = zeros(frameSize,1);
    else
        y(:,i) = u(:, index + 1); % add 1 for Matlab indexing
    end
end
